simulink model "ExtDem_CalcState"  (R2016b)
settings: configuration reference "CodeGenConfigSet" (kept outside this file)
values from neighbouring files (symbols this model uses):
  ExtDem_rAPPThresTrqDem_C = Calibration.Parameter    [init_ExtDem_CalcState.m]
  ExtDem_stMskFrzRls_C = Calibration.Parameter    [init_ExtDem_CalcState.m]
  ExtDem_swtAct_C = Calibration.Parameter    [init_ExtDem_CalcState.m]
undefined symbols (not defined in the file or in its folder): EISGov_num_conv, WESDem_State_conv
libraries: simulink x6, CXLib x5
settings Model: Creator=xuxingpei  LastModifiedBy=xuxingpei
settings ConfigSetRef: SourceLocation=Base Workspace

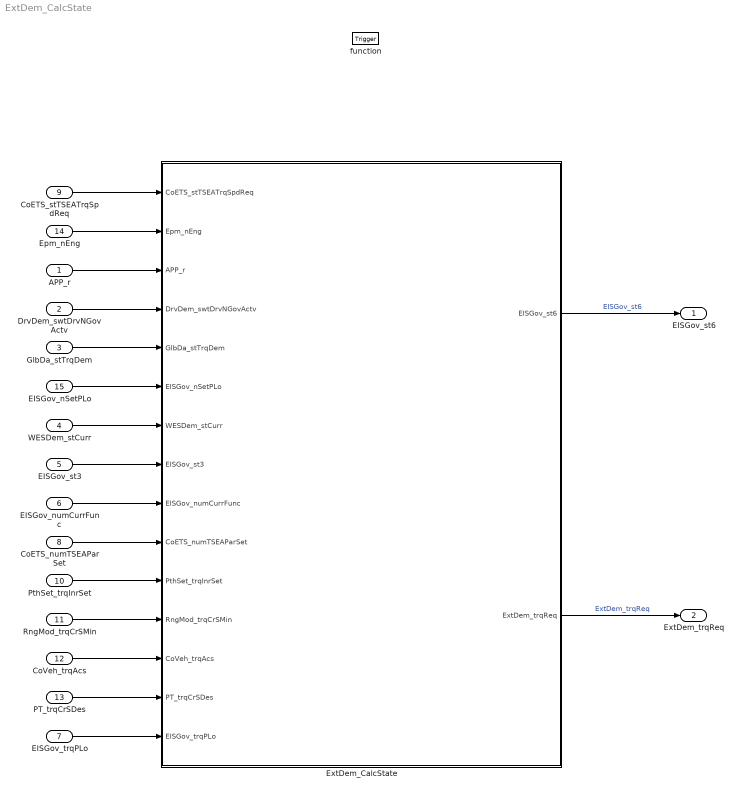
== system ExtDem_CalcState ==
  APP_r : Inport  Tag=%  Description=Acceleration pedal sensor 1 value after fault handling  OutMin=0  OutMax=100  OutDataTypeStr=Accpedal_rate
  DrvDem_swtDrvNGovActv : Inport  Description=Switch to activate DrvDem  Port=2  OutDataTypeStr=Enum: Switch_conv
  GlbDa_stTrqDem : Inport  Description=contains highest prior function with torque demand  Port=3  OutMin=0  OutMax=4294967295  OutDataTypeStr=State_uint32
  WESDem_stCurr : Inport  Description=Status of the working engine Speed Control  Port=4  OutDataTypeStr=Enum: WESDem_State_conv
  EISGov_st3 : Inport  Description=Status information of WESDem client  Port=5  OutMin=0  OutMax=2147483648  OutDataTypeStr=State_uint32
  EISGov_numCurrFunc : Inport  Description=Identification name / number of the currently active EISGov client, which determines the current controller parameters  Port=6  OutDataTypeStr=Enum: EISGov_num_conv
  EISGov_trqPLo : Inport  Tag=Nm  Description=P-component of the lower path  Port=7  OutMin=-3276.8  OutMax=3276.7  OutDataTypeStr=Trq_Nm
  CoETS_numTSEAParSet : Inport  Description=Number of requested parameter set for Engine speed governor  Port=8  OutMin=0  OutMax=255  OutDataTypeStr=State_uint8
  CoETS_stTSEATrqSpdReq : Inport  Description=Status of information about torque and speed intervention  Port=9  OutMin=0  OutMax=65535  OutDataTypeStr=State_uint16
  PthSet_trqInrSet : Inport  Tag=Nm  Description=Inner torque set value after monitoring limitation  Port=10  OutMin=-3000  OutMax=3276.7  OutDataTypeStr=Trq_Nm
  RngMod_trqCrSMin : Inport  Tag=Nm  Description=minimal crankshaft torque  Port=11  OutMin=-3276.8  OutMax=3276.7  OutDataTypeStr=Trq_Nm
  CoVeh_trqAcs : Inport  Tag=Nm  Description=message for demand of accessories  Port=12  OutMin=-3276.8  OutMax=3276.7  OutDataTypeStr=Trq_Nm
  PT_trqCrSDes : Inport  Tag=Nm  Description=Application parameter for requested propulsion torque to engine(crankshaft torque)  Port=13  OutMin=-3000  OutMax=3000  OutDataTypeStr=Trq_Nm
  Epm_nEng : Inport  Tag=rpm  Description=Engine speed  Port=14  OutMin=0  OutMax=6000  OutDataTypeStr=EngSpeed_rpm
  EISGov_nSetPLo : Inport  Tag=rpm  Description=Lower limit of the speed interval (set point speed) of the EISGov  Port=15  OutMin=0  OutMax=6000  OutDataTypeStr=EngSpeed_rpm
  function : TriggerPort  TriggerType=function-call  VariantControl=Variant
  ExtDem_CalcState : Subsystem
  EISGov_st6 : Outport  Description=Status information of ExtDem for EISGov and its clients  OutMin=0  OutMax=2147483648  OutDataTypeStr=State_uint32
  ExtDem_trqReq : Outport  Tag=Nm  Description=Torque intialization request of the EISGov External Intervention function  Port=2  OutMin=-3000  OutMax=3000  OutDataTypeStr=Trq_Nm
  wires:
  ExtDem_CalcState/1(EISGov_st6) -> EISGov_st6/1  "EISGov_st6"
  ExtDem_CalcState/2(ExtDem_trqReq) -> ExtDem_trqReq/1  "ExtDem_trqReq"
  APP_r/1 -> ExtDem_CalcState/3(APP_r)
  DrvDem_swtDrvNGovActv/1 -> ExtDem_CalcState/4(DrvDem_swtDrvNGovActv)
  GlbDa_stTrqDem/1 -> ExtDem_CalcState/5(GlbDa_stTrqDem)
  WESDem_stCurr/1 -> ExtDem_CalcState/7(WESDem_stCurr)
  EISGov_st3/1 -> ExtDem_CalcState/8(EISGov_st3)
  EISGov_numCurrFunc/1 -> ExtDem_CalcState/9(EISGov_numCurrFunc)
  CoETS_numTSEAParSet/1 -> ExtDem_CalcState/10(CoETS_numTSEAParSet)
  CoETS_stTSEATrqSpdReq/1 -> ExtDem_CalcState/1(CoETS_stTSEATrqSpdReq)
  PthSet_trqInrSet/1 -> ExtDem_CalcState/11(PthSet_trqInrSet)
  RngMod_trqCrSMin/1 -> ExtDem_CalcState/12(RngMod_trqCrSMin)
  CoVeh_trqAcs/1 -> ExtDem_CalcState/13(CoVeh_trqAcs)
  PT_trqCrSDes/1 -> ExtDem_CalcState/14(PT_trqCrSDes)
  Epm_nEng/1 -> ExtDem_CalcState/2(Epm_nEng)
  EISGov_nSetPLo/1 -> ExtDem_CalcState/6(EISGov_nSetPLo)
  EISGov_trqPLo/1 -> ExtDem_CalcState/15(EISGov_trqPLo)

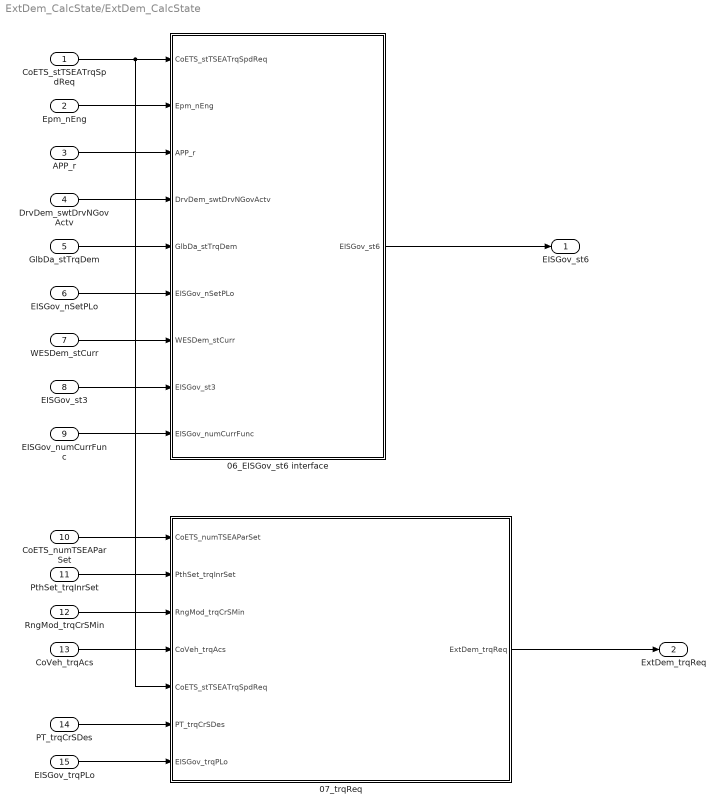
== system ExtDem_CalcState/ExtDem_CalcState ==
  CoETS_stTSEATrqSpdReq : Inport  Description=Status of information about torque and speed intervention  OutMin=0  OutMax=65535  OutDataTypeStr=State_uint16
  Epm_nEng : Inport  Tag=rpm  Description=Engine speed  Port=2  OutMin=0  OutMax=6000  OutDataTypeStr=EngSpeed_rpm
  APP_r : Inport  Tag=%  Description=Acceleration pedal sensor 1 value after fault handling  Port=3  OutMin=0  OutMax=100  OutDataTypeStr=Accpedal_rate
  DrvDem_swtDrvNGovActv : Inport  Description=Switch to activate DrvDem  Port=4  OutDataTypeStr=Enum: Switch_conv
  GlbDa_stTrqDem : Inport  Description=contains highest prior function with torque demand  Port=5  OutMin=0  OutMax=4294967295  OutDataTypeStr=State_uint32
  EISGov_nSetPLo : Inport  Port=6
  WESDem_stCurr : Inport  Description=Status of the working engine Speed Control  Port=7  OutDataTypeStr=Enum: WESDem_State_conv
  EISGov_st3 : Inport  Description=Status information of WESDem client  Port=8  OutMin=0  OutMax=2147483648  OutDataTypeStr=State_uint32
  EISGov_numCurrFunc : Inport  Description=Identification name / number of the currently active EISGov client, which determines the current controller parameters  Port=9  OutDataTypeStr=Enum: EISGov_num_conv
  CoETS_numTSEAParSet : Inport  Description=Number of requested parameter set for Engine speed governor  Port=10  OutMin=0  OutMax=255  OutDataTypeStr=State_uint8
  PthSet_trqInrSet : Inport  Tag=Nm  Description=Inner torque set value after monitoring limitation  Port=11  OutMin=-3000  OutMax=3276.7  OutDataTypeStr=Trq_Nm
  RngMod_trqCrSMin : Inport  Tag=Nm  Description=minimal crankshaft torque  Port=12  OutMin=-3276.8  OutMax=3276.7  OutDataTypeStr=Trq_Nm
  CoVeh_trqAcs : Inport  Tag=Nm  Description=message for demand of accessories  Port=13  OutMin=-3276.8  OutMax=3276.7  OutDataTypeStr=Trq_Nm
  PT_trqCrSDes : Inport  Tag=Nm  Description=Application parameter for requested propulsion torque to engine(crankshaft torque)  Port=14  OutMin=-3000  OutMax=3000  OutDataTypeStr=Trq_Nm
  EISGov_trqPLo : Inport  Tag=Nm  Description=P-component of the lower path  Port=15  OutMin=-3276.8  OutMax=3276.7  OutDataTypeStr=Trq_Nm
  "06_EISGov_st6 interface " : Subsystem
  07_trqReq : Subsystem
  EISGov_st6 : Outport  Description=Status information of ExtDem for EISGov and its clients
  ExtDem_trqReq : Outport  Tag=Nm  Description=Torque intialization request of the EISGov External Intervention function  Port=2
  wires:
  CoETS_stTSEATrqSpdReq/1 -> 07_trqReq/5(CoETS_stTSEATrqSpdReq), "06_EISGov_st6 interface "/1(CoETS_stTSEATrqSpdReq)
  Epm_nEng/1 -> "06_EISGov_st6 interface "/2(Epm_nEng)
  PT_trqCrSDes/1 -> 07_trqReq/6(PT_trqCrSDes)
  CoVeh_trqAcs/1 -> 07_trqReq/4(CoVeh_trqAcs)
  RngMod_trqCrSMin/1 -> 07_trqReq/3(RngMod_trqCrSMin)
  DrvDem_swtDrvNGovActv/1 -> "06_EISGov_st6 interface "/4(DrvDem_swtDrvNGovActv)
  EISGov_nSetPLo/1 -> "06_EISGov_st6 interface "/6(EISGov_nSetPLo)
  EISGov_numCurrFunc/1 -> "06_EISGov_st6 interface "/9(EISGov_numCurrFunc)
  CoETS_numTSEAParSet/1 -> 07_trqReq/1(CoETS_numTSEAParSet)
  APP_r/1 -> "06_EISGov_st6 interface "/3(APP_r)
  PthSet_trqInrSet/1 -> 07_trqReq/2(PthSet_trqInrSet)
  07_trqReq/1(ExtDem_trqReq) -> ExtDem_trqReq/1
  "06_EISGov_st6 interface "/1(EISGov_st6) -> EISGov_st6/1
  GlbDa_stTrqDem/1 -> "06_EISGov_st6 interface "/5(GlbDa_stTrqDem)
  EISGov_st3/1 -> "06_EISGov_st6 interface "/8(EISGov_st3)
  WESDem_stCurr/1 -> "06_EISGov_st6 interface "/7(WESDem_stCurr)
  EISGov_trqPLo/1 -> 07_trqReq/7(EISGov_trqPLo)

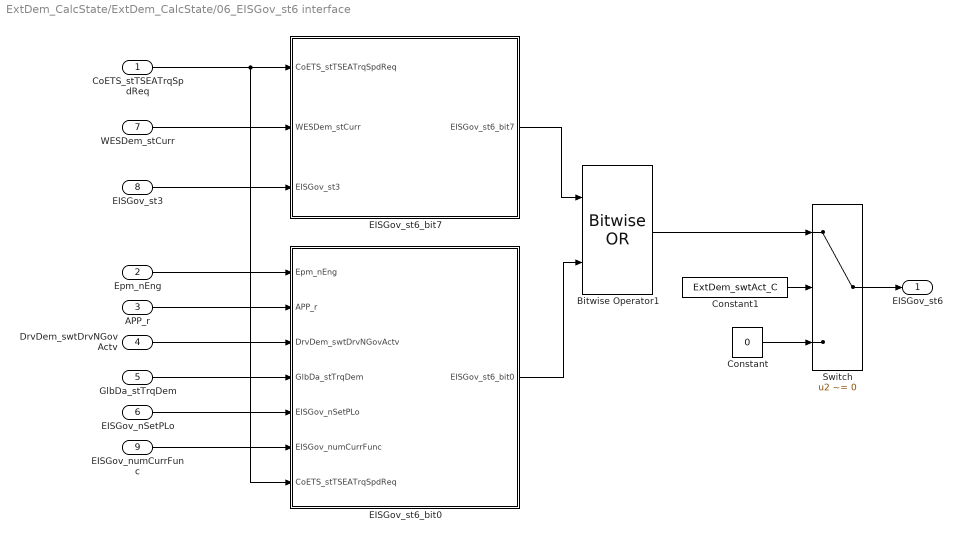
== system ExtDem_CalcState/ExtDem_CalcState/06_EISGov_st6 interface  ==
  CoETS_stTSEATrqSpdReq : Inport  Description=Status of information about torque and speed intervention  OutMin=0  OutMax=65535  OutDataTypeStr=State_uint16
  Epm_nEng : Inport  Tag=rpm  Description=Engine speed  Port=2  OutMin=0  OutMax=6000  OutDataTypeStr=EngSpeed_rpm
  APP_r : Inport  Tag=%  Description=Acceleration pedal sensor 1 value after fault handling  Port=3  OutMin=0  OutMax=100  OutDataTypeStr=Accpedal_rate
  DrvDem_swtDrvNGovActv : Inport  Description=Switch to activate DrvDem  Port=4  OutDataTypeStr=Enum: Switch_conv
  GlbDa_stTrqDem : Inport  Description=contains highest prior function with torque demand  Port=5  OutMin=0  OutMax=4294967295  OutDataTypeStr=State_uint32
  EISGov_nSetPLo : Inport  Tag=rpm  Description=Lower limit of the speed interval (set point speed) of the EISGov  Port=6  OutMin=0  OutMax=6000  OutDataTypeStr=EngSpeed_rpm
  WESDem_stCurr : Inport  Description=Status of the working engine Speed Control  Port=7  OutDataTypeStr=Enum: WESDem_State_conv
  EISGov_st3 : Inport  Description=Status information of WESDem client  Port=8  OutMin=0  OutMax=2147483648  OutDataTypeStr=State_uint32
  EISGov_numCurrFunc : Inport  Description=Identification name / number of the currently active EISGov client, which determines the current controller parameters  Port=9  OutDataTypeStr=Enum: EISGov_num_conv
  Bitwise Operator1 : simulink/Logic and Bit Operations/Bitwise Operator  logicop=OR  UseBitMask=off  NumInputPorts=2  BitMask=bin2dec('11011001')  BitMaskRealWorld=Stored Integer
  Constant : Constant  Value=0  OutDataTypeStr=uint32
  Constant1 : Constant  Value=ExtDem_swtAct_C
  EISGov_st6_bit0 : Subsystem
  EISGov_st6_bit7 : Subsystem
  Switch : Switch  Criteria=u2 ~= 0  InputSameDT=on
  EISGov_st6 : Outport  Description=Status information of ExtDem for EISGov and its clients  OutMin=0  OutMax=2147483648  OutDataTypeStr=State_uint32
  wires:
  Bitwise Operator1/1 -> Switch/1
  Epm_nEng/1 -> EISGov_st6_bit0/1(Epm_nEng)
  APP_r/1 -> EISGov_st6_bit0/2(APP_r)
  DrvDem_swtDrvNGovActv/1 -> EISGov_st6_bit0/3(DrvDem_swtDrvNGovActv)
  GlbDa_stTrqDem/1 -> EISGov_st6_bit0/4(GlbDa_stTrqDem)
  EISGov_nSetPLo/1 -> EISGov_st6_bit0/5(EISGov_nSetPLo)
  EISGov_st6_bit0/1(EISGov_st6_bit0) -> Bitwise Operator1/2
  EISGov_st3/1 -> EISGov_st6_bit7/3(EISGov_st3)
  WESDem_stCurr/1 -> EISGov_st6_bit7/2(WESDem_stCurr)
  CoETS_stTSEATrqSpdReq/1 -> EISGov_st6_bit0/7(CoETS_stTSEATrqSpdReq), EISGov_st6_bit7/1(CoETS_stTSEATrqSpdReq)
  EISGov_st6_bit7/1(EISGov_st6_bit7) -> Bitwise Operator1/1
  Switch/1 -> EISGov_st6/1
  Constant/1 -> Switch/3
  Constant1/1 -> Switch/2
  EISGov_numCurrFunc/1 -> EISGov_st6_bit0/6(EISGov_numCurrFunc)

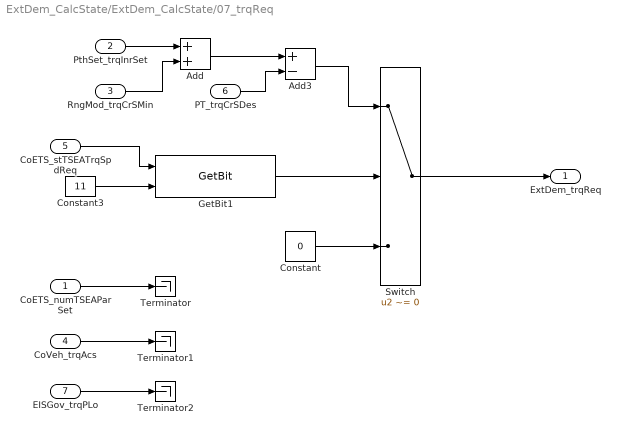
== system ExtDem_CalcState/ExtDem_CalcState/07_trqReq ==
  CoETS_numTSEAParSet : Inport  Description=Number of requested parameter set for Engine speed governor  OutMin=0  OutMax=255  OutDataTypeStr=State_uint8
  PthSet_trqInrSet : Inport  Tag=Nm  Description=Inner torque set value after monitoring limitation  Port=2  OutMin=-3000  OutMax=3276.7  OutDataTypeStr=Trq_Nm
  RngMod_trqCrSMin : Inport  Port=3
  CoVeh_trqAcs : Inport  Tag=Nm  Description=message for demand of accessories  Port=4  OutMin=-3276.8  OutMax=3276.7  OutDataTypeStr=Trq_Nm
  CoETS_stTSEATrqSpdReq : Inport  Description=Status of information about torque and speed intervention  Port=5  OutMin=0  OutMax=65535  OutDataTypeStr=State_uint16
  PT_trqCrSDes : Inport  Port=6
  EISGov_trqPLo : Inport  Tag=Nm  Description=P-component of the lower path  Port=7  OutMin=-3276.8  OutMax=3276.7  OutDataTypeStr=Trq_Nm
  Add : Sum  SaturateOnIntegerOverflow=on
  Add3 : Sum  Inputs=+-  SaturateOnIntegerOverflow=on
  Constant : Constant  Value=0  OutDataTypeStr=Inherit: Inherit via back propagation
  Constant3 : Constant  Value=11  OutDataTypeStr=Inherit: Inherit via back propagation
  GetBit1 : CXLib/GetBit  dataTypeString=uint16  dataLength=0
      settings: AttributesFormatString=Get bit from %<dataTypeString>
  Switch : Switch  Criteria=u2 ~= 0
  Terminator : Terminator
  Terminator1 : Terminator
  Terminator2 : Terminator
  ExtDem_trqReq : Outport  Tag=Nm  Description=Torque intialization request of the EISGov External Intervention function  OutMin=-3000  OutMax=3000  OutDataTypeStr=Trq_Nm
  wires:
  Switch/1 -> ExtDem_trqReq/1
  PthSet_trqInrSet/1 -> Add/1
  RngMod_trqCrSMin/1 -> Add/2
  Constant3/1 -> GetBit1/2
  CoETS_numTSEAParSet/1 -> Terminator/1
  Add/1 -> Add3/1
  Add3/1 -> Switch/1
  PT_trqCrSDes/1 -> Add3/2
  CoVeh_trqAcs/1 -> Terminator1/1
  CoETS_stTSEATrqSpdReq/1 -> GetBit1/1
  GetBit1/1 -> Switch/2
  Constant/1 -> Switch/3
  EISGov_trqPLo/1 -> Terminator2/1

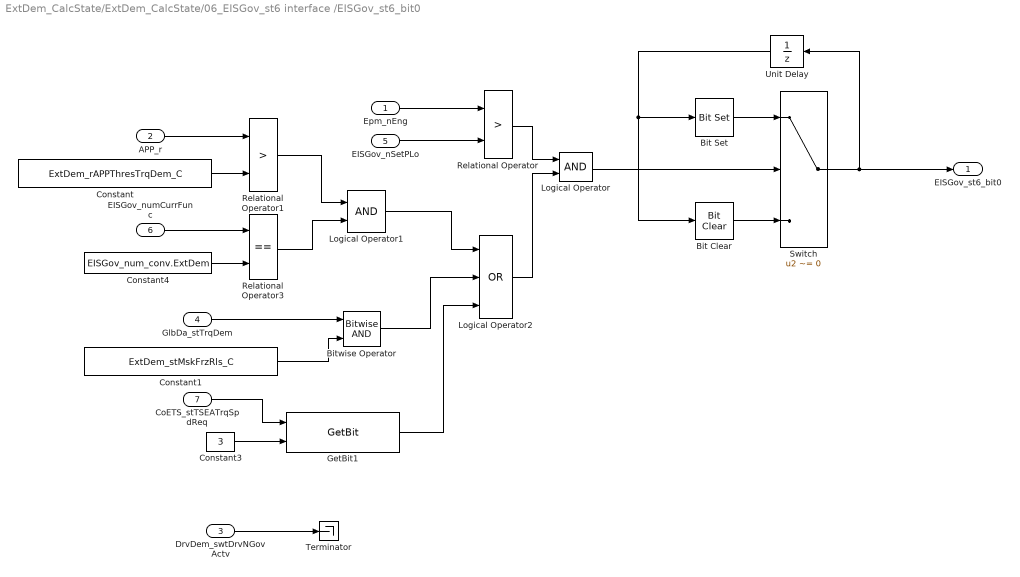
== system ExtDem_CalcState/ExtDem_CalcState/06_EISGov_st6 interface /EISGov_st6_bit0 ==
  Epm_nEng : Inport  Tag=rpm  Description=Engine speed  OutMin=0  OutMax=6000  OutDataTypeStr=EngSpeed_rpm
  APP_r : Inport  Tag=%  Description=Acceleration pedal sensor 1 value after fault handling  Port=2  OutMin=0  OutMax=100  OutDataTypeStr=Accpedal_rate
  DrvDem_swtDrvNGovActv : Inport  Description=Switch to activate DrvDem  Port=3  OutDataTypeStr=Enum: Switch_conv
  GlbDa_stTrqDem : Inport  Description=contains highest prior function with torque demand  Port=4  OutMin=0  OutMax=4294967295  OutDataTypeStr=State_uint32
  EISGov_nSetPLo : Inport  Tag=rpm  Description=Lower limit of the speed interval (set point speed) of the EISGov  Port=5  OutMin=0  OutMax=6000  OutDataTypeStr=EngSpeed_rpm
  EISGov_numCurrFunc : Inport  Port=6
  CoETS_stTSEATrqSpdReq : Inport  Description=Status of information about torque and speed intervention  Port=7  OutMin=0  OutMax=65535  OutDataTypeStr=State_uint16
  Bit Clear : simulink/Logic and Bit Operations/Bit Clear  iBit=0
  Bit Set : simulink/Logic and Bit Operations/Bit Set  iBit=0
  Bitwise Operator : simulink/Logic and Bit Operations/Bitwise Operator  logicop=AND  UseBitMask=off  NumInputPorts=2  BitMask=bin2dec('11011001')  BitMaskRealWorld=Stored Integer
  Constant : Constant  Value=ExtDem_rAPPThresTrqDem_C
  Constant1 : Constant  Value=ExtDem_stMskFrzRls_C
  Constant3 : Constant  Value=3  OutDataTypeStr=Inherit: Inherit via back propagation
  Constant4 : Constant  Value=EISGov_num_conv.ExtDem
  GetBit1 : CXLib/GetBit  dataTypeString=uint16  dataLength=0
      settings: AttributesFormatString=Get bit from %<dataTypeString>
  Logical Operator : Logic  AllPortsSameDT=off  OutDataTypeStr=boolean
  Logical Operator1 : Logic  AllPortsSameDT=off  OutDataTypeStr=boolean
  Logical Operator2 : Logic  Operator=OR  Inputs=3  AllPortsSameDT=off  OutDataTypeStr=boolean
  Relational Operator : RelationalOperator  Operator=>  OutDataTypeStr=boolean  RndMeth=Simplest
  Relational Operator1 : RelationalOperator  Operator=>  OutDataTypeStr=boolean  RndMeth=Simplest
  Relational Operator3 : RelationalOperator  Operator===  OutDataTypeStr=boolean  RndMeth=Nearest  InputSameDT=on
  Switch : Switch  Criteria=u2 ~= 0  InputSameDT=on
  Terminator : Terminator
  Unit Delay : UnitDelay  SampleTime=-1
      settings: AttributesFormatString=InitialValue=%<InitialCondition>
  EISGov_st6_bit0 : Outport
  wires:
  Switch/1 -> EISGov_st6_bit0/1, Unit Delay/1
  Constant1/1 -> Bitwise Operator/2
  Bitwise Operator/1 -> Logical Operator2/2
  Relational Operator/1 -> Logical Operator/1
  Logical Operator2/1 -> Logical Operator/2
  Logical Operator1/1 -> Logical Operator2/1
  EISGov_nSetPLo/1 -> Relational Operator/2
  Epm_nEng/1 -> Relational Operator/1
  Constant/1 -> Relational Operator1/2
  Relational Operator1/1 -> Logical Operator1/1
  GlbDa_stTrqDem/1 -> Bitwise Operator/1
  APP_r/1 -> Relational Operator1/1
  Logical Operator/1 -> Switch/2
  Unit Delay/1 -> Bit Clear/1, Bit Set/1
  Bit Set/1 -> Switch/1
  Bit Clear/1 -> Switch/3
  EISGov_numCurrFunc/1 -> Relational Operator3/1
  Constant4/1 -> Relational Operator3/2
  Relational Operator3/1 -> Logical Operator1/2
  GetBit1/1 -> Logical Operator2/3
  DrvDem_swtDrvNGovActv/1 -> Terminator/1
  Constant3/1 -> GetBit1/2
  CoETS_stTSEATrqSpdReq/1 -> GetBit1/1

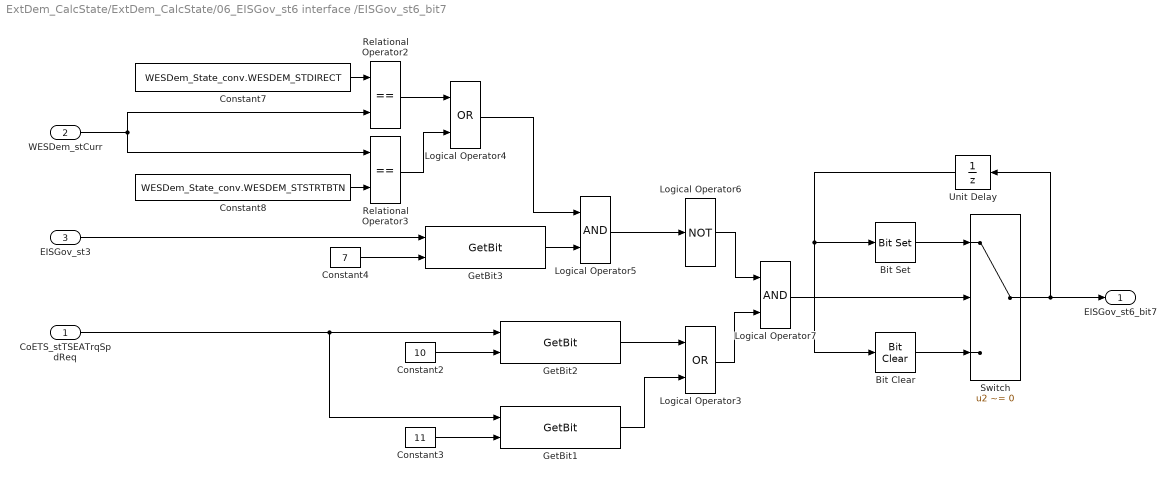
== system ExtDem_CalcState/ExtDem_CalcState/06_EISGov_st6 interface /EISGov_st6_bit7 ==
  CoETS_stTSEATrqSpdReq : Inport  Description=Status of information about torque and speed intervention  OutMin=0  OutMax=65535  OutDataTypeStr=State_uint16
  WESDem_stCurr : Inport  Description=Status of the working engine Speed Control  Port=2  OutDataTypeStr=Enum: WESDem_State_conv
  EISGov_st3 : Inport  Description=Status information of WESDem client  Port=3  OutMin=0  OutMax=2147483648  OutDataTypeStr=State_uint32
  Bit Clear : simulink/Logic and Bit Operations/Bit Clear  iBit=7
  Bit Set : simulink/Logic and Bit Operations/Bit Set  iBit=7
  Constant2 : Constant  Value=10  OutDataTypeStr=Inherit: Inherit via back propagation
  Constant3 : Constant  Value=11  OutDataTypeStr=Inherit: Inherit via back propagation
  Constant4 : Constant  Value=7  OutDataTypeStr=Inherit: Inherit via back propagation
  Constant7 : Constant  Value=WESDem_State_conv.WESDEM_STDIRECT  OutDataTypeStr=Inherit: Inherit via back propagation
  Constant8 : Constant  Value=WESDem_State_conv.WESDEM_STSTRTBTN  OutDataTypeStr=Inherit: Inherit via back propagation
  GetBit1 : CXLib/GetBit  dataTypeString=uint16  dataLength=0
      settings: AttributesFormatString=Get bit from %<dataTypeString>
  GetBit2 : CXLib/GetBit  dataTypeString=uint16  dataLength=0
      settings: AttributesFormatString=Get bit from %<dataTypeString>
  GetBit3 : CXLib/GetBit  dataTypeString=uint32  dataLength=0
      settings: AttributesFormatString=Get bit from %<dataTypeString>
  Logical Operator3 : Logic  Operator=OR  OutDataTypeStr=boolean
  Logical Operator4 : Logic  Operator=OR  OutDataTypeStr=boolean
  Logical Operator5 : Logic  OutDataTypeStr=boolean
  Logical Operator6 : Logic  Operator=NOT  OutDataTypeStr=boolean
  Logical Operator7 : Logic  OutDataTypeStr=boolean
  Relational Operator2 : RelationalOperator  Operator===  OutDataTypeStr=boolean  RndMeth=Simplest  InputSameDT=on
  Relational Operator3 : RelationalOperator  Operator===  OutDataTypeStr=boolean  RndMeth=Simplest  InputSameDT=on
  Switch : Switch  Criteria=u2 ~= 0  InputSameDT=on
  Unit Delay : UnitDelay  SampleTime=-1
      settings: AttributesFormatString=InitialValue=%<InitialCondition>
  EISGov_st6_bit7 : Outport
  wires:
  Constant2/1 -> GetBit2/2
  GetBit1/1 -> Logical Operator3/2
  GetBit3/1 -> Logical Operator5/2
  GetBit2/1 -> Logical Operator3/1
  Logical Operator5/1 -> Logical Operator6/1
  Logical Operator4/1 -> Logical Operator5/1
  Logical Operator7/1 -> Switch/2
  Unit Delay/1 -> Bit Clear/1, Bit Set/1
  Bit Set/1 -> Switch/1
  Logical Operator6/1 -> Logical Operator7/1
  Switch/1 -> EISGov_st6_bit7/1, Unit Delay/1
  WESDem_stCurr/1 -> Relational Operator3/1, Relational Operator2/2
  Constant3/1 -> GetBit1/2
  CoETS_stTSEATrqSpdReq/1 -> GetBit1/1, GetBit2/1
  Logical Operator3/1 -> Logical Operator7/2
  Bit Clear/1 -> Switch/3
  Relational Operator2/1 -> Logical Operator4/1
  Relational Operator3/1 -> Logical Operator4/2
  Constant8/1 -> Relational Operator3/2
  Constant7/1 -> Relational Operator2/1
  EISGov_st3/1 -> GetBit3/1
  Constant4/1 -> GetBit3/2
